simulink model "final_p4_ssKF"  (R2021a)
settings: Solver=VariableStepAuto  StartTime=0.0  StopTime=30  RelTol=1e-8
values from neighbouring files (symbols this model uses):
  Akf = A - L*C    [final_p4.m]
  As = A    [final_p4.m]
  Bkf = [L, B1]    [final_p4.m]
  Bs = [B0, B1]    [final_p4.m]
  C = {}    [final_p2i.m]    (also in final_p2ii.m; final_p4.m = [1 0 0 0; 0 0 1 0])
  Ckf = eye(4)    [final_p4.m]
  Cs = eye(4)    [final_p4.m]
  D = {}    [final_p2i.m]    (also in final_p2ii.m; final_p4.m = [0.25 0; 0 0.05])
  Dkf = zeros(size(Ckf,1), size(Bkf,2))    [final_p4.m]
  Ds = zeros(size(Cs,1), size(Bs,2))    [final_p4.m]
  K = lqr(A, B1, diag([1,2,4,2]), diag([0.1]))    [final_p4.m]
libraries: simulink x4
settings Model: Creator=Tomo  LastModifiedBy=Tomo

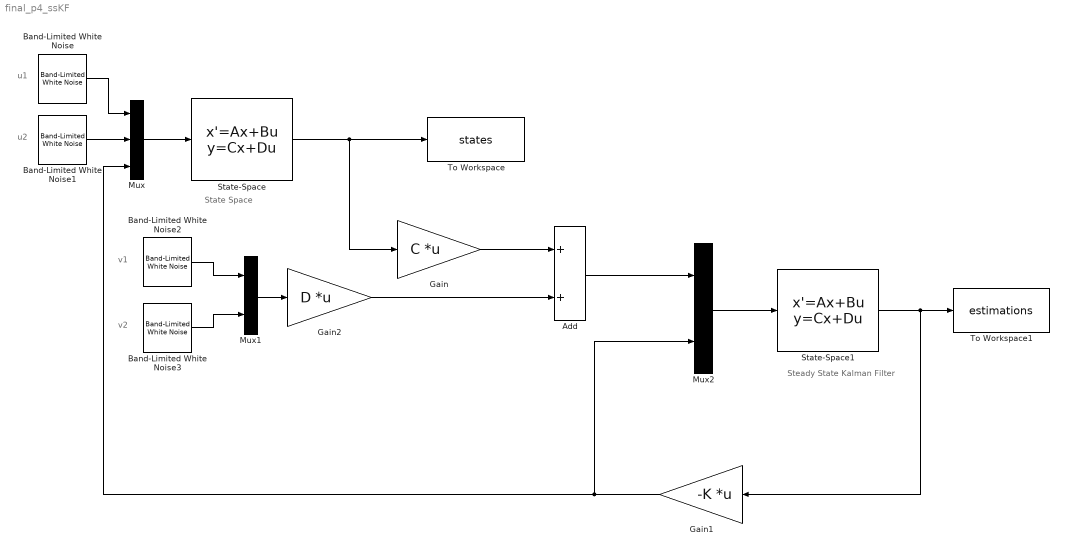
== system final_p4_ssKF ==
  note: State Space
  note: u1
  note: u2
  note: v2
  note: v1
  note: Steady State
      | Kalman Filter
  Add : Sum
  Band-Limited White Noise : simulink/Sources/Band-Limited White Noise  Cov=[0.1]  Ts=0.1  seed=[23341]
  Band-Limited White Noise1 : simulink/Sources/Band-Limited White Noise  Cov=[0.1]  Ts=0.1  seed=[23342]
  Band-Limited White Noise2 : simulink/Sources/Band-Limited White Noise  Cov=[0.1]  Ts=0.1  seed=[23343]
  Band-Limited White Noise3 : simulink/Sources/Band-Limited White Noise  Cov=[0.1]  Ts=0.1  seed=[23344]
  Gain : Gain  Gain=C  Multiplication=Matrix(K*u)
  Gain1 : Gain  Gain=-K  Multiplication=Matrix(K*u)
  Gain2 : Gain  Gain=D  Multiplication=Matrix(K*u)
  Mux : Mux  Inputs=3
  Mux1 : Mux  Inputs=2
  Mux2 : Mux  Inputs=2
  State-Space : StateSpace  A=As  B=Bs  C=Cs  D=Ds  InitialCondition=0
  State-Space1 : StateSpace  A=Akf  B=Bkf  C=Ckf  D=Dkf  InitialCondition=0
  To Workspace : ToWorkspace  VariableName=states  SaveFormat=Structure With Time  SampleTime=-1
  To Workspace1 : ToWorkspace  VariableName=estimations  SaveFormat=Structure With Time  SampleTime=-1
  wires:
  Band-Limited White Noise/1 -> Mux/1
  Band-Limited White Noise1/1 -> Mux/2
  Band-Limited White Noise3/1 -> Mux1/2
  Band-Limited White Noise2/1 -> Mux1/1
  State-Space/1 -> To Workspace/1, Gain/1
  Gain/1 -> Add/1
  Mux1/1 -> Gain2/1
  Add/1 -> Mux2/1
  Mux2/1 -> State-Space1/1
  Mux/1 -> State-Space/1
  Gain1/1 -> Mux2/2, Mux/3
  Gain2/1 -> Add/2
  State-Space1/1 -> To Workspace1/1, Gain1/1
